simulink library "elvio"  (R2017a)
settings: Solver=VariableStepAuto  StartTime=0.0  StopTime=10.0  RelTol=1e-3
values from neighbouring files (symbols this model uses):
  Ts = 1    [dynorun.m]
  v = [v1;v2]    [elvio_plot_scatter.m]
undefined symbols (not defined in the file or in its folder): dm, elvio_tag_from, elvio_tag_goto, energy, F, Fmax, Fmin, Freq, m, request, speed, vcur
undefined symbols (not defined in the file): containers, torque
libraries: elvio x92, simulink x6
(part 1 of 2)
settings Model: Creator=elts2  LastModifiedBy=thomas

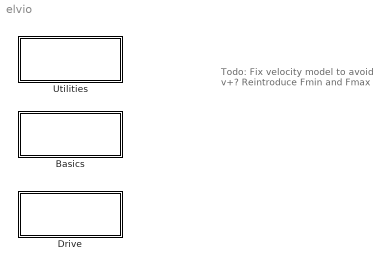
== system elvio ==
  note: Todo:
      | Fix velocity model to avoid v+?
      | Reintroduce Fmin and Fmax
  Basics : Subsystem
  Drive : Subsystem
  Utilities : Subsystem

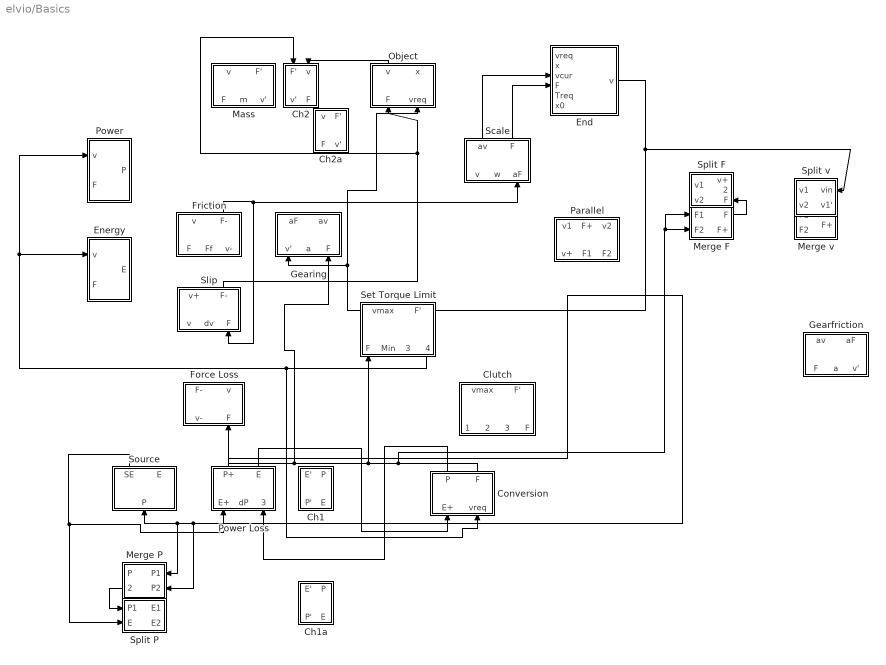
== system elvio/Basics ==
  Ch1 : Subsystem
  Ch1a : Subsystem
  Ch2 : Subsystem
  Ch2a : Subsystem
  Clutch : Subsystem
  Conversion : Subsystem
  End : Subsystem
  Energy : Subsystem
  Force Loss : Subsystem  mask{factor=0.1}
      mask prompts: factor "Loss Factor:"
  Friction : Subsystem
  Gearfriction : Subsystem
  Gearing : Subsystem
  Mass : Subsystem
  Merge F : Subsystem
  Merge P : Subsystem
  Merge v : Subsystem
  Object : Subsystem
  Parallel : Subsystem
  Power : Subsystem
  Power Loss : Subsystem
  Scale : Subsystem
  Set Torque Limit : Subsystem
  Slip : Subsystem
  Source : Subsystem
  Split F : Subsystem
  Split P : Subsystem
  Split v : Subsystem
  wires:
  Conversion/1(P) -> Power Loss/3(Preq)
  End/1(v) -> Split v/1(vin), Conversion/2(vreq), Power/1(v), Energy/1(v), Object/2(vreq), Gearing/1(v')
  Power Loss/1(P+) -> Merge P/2(P2), Merge P/1(P1), Source/1(P)
  Source/1(SE) -> Split P/2(E), Power Loss/1(E+)
  Conversion/2(F) -> Merge F/1(F1), Merge F/2(F2), Set Torque Limit/1(F), Force Loss/2(F), Gearing/3(F)
  Friction/2(F-) -> Scale/3(aF), Slip/3(F)
  Scale/1(av) -> End/3(vcur)
  Scale/2(F) -> End/4(F)
  Slip/2(F-) -> Ch2/1(F'), Object/1(F)
  Merge F/1(F) -> Split F/3(F)
  Power Loss/2(E) -> Conversion/1(E+)
  Object/1(v) -> Ch2/2(v)
  Merge P/2(P1'1) -> Split P/1(P1)

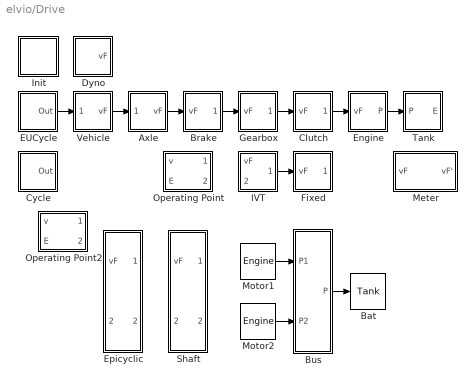
== system elvio/Drive ==
  Axle : Subsystem  InitFcn=|  mask{radius=0.3, ratio=4, factor=0.1, FromTag1=Vehicle1, GotoTag1=F}
      | elvio_tag_from([1]);
      | elvio_tag_goto([1]);
      mask prompts: radius "Tyre Radius (in m):"; ratio "Final Drive (ratio):"; factor "Loss Factor (factor):"; FromTag1 "Simulink:blkprm_prompts:FromGotoTag"; GotoTag1 "Simulink:blkprm_prompts:GotoTag"
      mask TypeOptions factor: Force Loss/factor
      mask TypeOptions FromTag1: From/GotoTag
      mask TypeOptions GotoTag1: Goto/GotoTag
  Bat : elvio/Drive/Tank  GotoTag1=F
  Brake : Subsystem  InitFcn=|  mask(Brake){Tbrake=5000, FromTag1=Vehicle1, GotoTag1=F}
      | elvio_tag_from([1]);
      | elvio_tag_goto([1]);
      mask prompts: Tbrake "Available Braking Torque (in Nm):"; FromTag1 "Simulink:blkprm_prompts:FromGotoTag"; GotoTag1 "Simulink:blkprm_prompts:GotoTag"
      mask help: This block adds braking torque when the powertrain cannot provide enough braking.
      mask TypeOptions FromTag1: From/GotoTag
      mask TypeOptions GotoTag1: Goto/GotoTag
  Bus : Subsystem  InitFcn=|  mask(DC Bus){GotoTag1=F, GotoTag2=E2, FromTag1=E}
      | elvio_tag_from([1]);
      | elvio_tag_goto([1 2]);
      mask prompts: GotoTag1 "Simulink:blkprm_prompts:GotoTag"; GotoTag2 "Simulink:blkprm_prompts:GotoTag"; FromTag1 "Simulink:blkprm_prompts:FromGotoTag"
      mask help: The DC bus connects two drives to one DC source.
      mask TypeOptions GotoTag1: Goto1/GotoTag
      mask TypeOptions GotoTag2: Goto2/GotoTag
      mask TypeOptions FromTag1: From1/GotoTag
  Clutch : Subsystem  InitFcn=|  mask(Clutch){speed=70, FromTag1=Vehicle1, GotoTag1=F}
      | elvio_tag_from([1]);
      | elvio_tag_goto([1]);
      mask prompts: speed "Minimum Speed (rad/s):"; FromTag1 "Simulink:blkprm_prompts:FromGotoTag"; GotoTag1 "Simulink:blkprm_prompts:GotoTag"
      mask help: This block enforces a minimal engine speed, simulating a slipping clutch when necessary.
      mask TypeOptions FromTag1: From/GotoTag
      mask TypeOptions GotoTag1: Goto/GotoTag
  Cycle : Subsystem  mask(Global Cycle){data=elvio_cycle_cadc_mw150()}
      mask prompts: data "Cycle:"
      mask help: This block generates one of the global cycles. Tolerances and gear information are reconstructed based on the approach used for NEDC.
      mask TypeOptions data: elvio_cycle_cadc_mw150() | elvio_cycle_cadc_rural() | elvio_cycle_cadc_urban() | elvio_cycle_cadc_urm150() | elvio_cycle_us_ftp75() | elvio_cycle_us_us06() | elvio_cycle_wltp_3b()
  Dyno : Subsystem  InitFcn=elvio_tag_from([1]);  mask{speed=speed, torque=torque, FromTag1=Dyno1}
      mask prompts: FromTag1 "Simulink:blkprm_prompts:FromGotoTag"
      mask TypeOptions FromTag1: From/GotoTag
  EUCycle : Subsystem  mask(European Cycle){data=elvio_cycle_nedc()}
      mask prompts: data "Cycle:"
      mask help: This block generates one of the European Cycles according to Regulation UNECE R83, including permissible tolerances and gear information.
      mask TypeOptions data: elvio_cycle_nedc() | elvio_cycle_ece15() | elvio_cycle_eudc()
  Engine : Subsystem  InitFcn=|  mask(Loss Model){Tmax=110, Tmin=0, Tfrict=16, Ploss=800, lossf=0.8, lossnorm=125e3, lossR=0.25, FromTag1=E, GotoTag1=F}
      | elvio_tag_from([1]);
      | elvio_tag_goto([1]);
      mask prompts: Tmax "Max Torque:"; Tmin "Min Torque:"; Tfrict "Friction Torque (Nm):"; Ploss "Power Loss (W):"; lossf "Loss Factor (factor):"; lossnorm "Square Loss Normal (W):"; lossR "Slip Loss (rad/Nms):"; FromTag1 "Simulink:blkprm_prompts:FromGotoTag"; GotoTag1 "Simulink:blkprm_prompts:GotoTag"
      mask help: A simple parametric engine or motor model based on 5 loss models.
      mask Help:
      | The five loss models are:
      |  * constant friction torque
      |  * constant power loss
      |  * constant efficiency loss
      |  * slip like loss (damping)
      |  * square of the power loss, defined using the nomalized power where the loss equalls the full power
      | 
      | To create a model with twice the torque, the friction, power loss, and square loss have to doubled, and the slip damping has to be halved.
      | 
      | To create a model with twice the speed, the power loss, the slip damping, and the square power have to be doubled.
      mask TypeOptions FromTag1: From/GotoTag
      mask TypeOptions GotoTag1: Goto/GotoTag
  Epicyclic : Subsystem  InitFcn=|  mask(Epicyclic Gearbox){a=0.3, FromTag1=E, FromTag2=F2, GotoTag1=F}
      | elvio_tag_from([1 2]);
      | elvio_tag_goto([1]);
      mask prompts: a "Sun to Ring Ratio (factor):"; FromTag1 "Simulink:blkprm_prompts:FromGotoTag"; FromTag2 "Simulink:blkprm_prompts:FromGotoTag"; GotoTag1 "Simulink:blkprm_prompts:GotoTag"
      mask help:
      | Model of an epicyclic gearbox (or velocity summing junction).
      |
      | It combines the speed of two prime movers, and splits the torque evenly according to the ratio.
      |
      | Rc is the relocity reference for the carrier vFc.
      mask TypeOptions FromTag1: From1/GotoTag
      mask TypeOptions FromTag2: From2/GotoTag
      mask TypeOptions GotoTag1: Goto/GotoTag
  Fixed : Subsystem  InitFcn=|  mask(Fixed Gear){gear=2, factor=0.1, FromTag1=E, GotoTag1=F}
      | elvio_tag_from([1]);
      | elvio_tag_goto([1]);
      mask prompts: gear "Gearing (ratio):"; factor "Loss Factor (factor):"; FromTag1 "Simulink:blkprm_prompts:FromGotoTag"; GotoTag1 "Simulink:blkprm_prompts:GotoTag"
      mask help: Model of a fixed gear with constant efficiency.
      mask TypeOptions factor: Force Loss/factor
      mask TypeOptions FromTag1: From/GotoTag
      mask TypeOptions GotoTag1: Goto/GotoTag
  Gearbox : Subsystem  InitFcn=|  mask(Manual Gearbox){gears=[4 2.5 1.8 1.2 0.9 0.9], factor=0.1, FromTag1=Gearbox1, GotoTag1=Brake1}
      | elvio_tag_from([1]);
      | elvio_tag_goto([1]);
      mask prompts: gears "Gears (vector):"; factor "Loss Factor (factor):"; FromTag1 "Simulink:blkprm_prompts:FromGotoTag"; GotoTag1 "Simulink:blkprm_prompts:GotoTag"
      mask help: This block is a manual gearbox. It applies to gear chosen by the cycle.
      mask TypeOptions factor: Force Loss/factor
      mask TypeOptions FromTag1: From/GotoTag
      mask TypeOptions GotoTag1: Goto/GotoTag
  IVT : Subsystem  InitFcn=|  mask{factor=0.1, FromTag1=E, GotoTag1=F}
      | elvio_tag_from([1]);
      | elvio_tag_goto([1]);
      mask prompts: factor "Loss Factor:"; FromTag1 "Simulink:blkprm_prompts:FromGotoTag"; GotoTag1 "Simulink:blkprm_prompts:GotoTag"
      mask TypeOptions factor: Force Loss/factor
      mask TypeOptions FromTag1: From/GotoTag
      mask TypeOptions GotoTag1: Goto/GotoTag
  Init : Subsystem  InitFcn=|  mask(Initialization Block){Ts0=1}
      | if ~exist('Ts')
      |     Ts = Ts0;
      | end
      | 
      | if ~exist('handle')
      |     handle = struct();
      | end
      mask prompts: Ts0 "Sample Time:"
      mask help: Initialize the Elvio library. This block sets the sampling time. It needs to be present in every Elvio model.
  Meter : Subsystem  InitFcn=|  mask(Energy Meter){FromTag1=E, GotoTag1=F}
      | elvio_tag_from([1]);
      | elvio_tag_goto([1]);
      mask prompts: FromTag1 "Simulink:blkprm_prompts:FromGotoTag"; GotoTag1 "Simulink:blkprm_prompts:GotoTag"
      mask help: Displays how much energy has flown through this connection so far, in J.
      mask TypeOptions FromTag1: From/GotoTag
      mask TypeOptions GotoTag1: Goto/GotoTag
  Motor1 : elvio/Drive/Engine  Tmax=60  Tmin=0  Tfrict=0.2  Ploss=100  lossf=0.01  lossnorm=2e6  lossR=0.05  FromTag1=E  GotoTag1=F
  Motor2 : elvio/Drive/Engine  Tmax=60  Tmin=-60  Tfrict=1  Ploss=200  lossf=0.01  lossnorm=1e6  lossR=0.1  FromTag1=E  GotoTag1=F
  Operating Point : Subsystem  mask{a=0.4, T=1000, Pk=0.5, Pbias=10e3, Pmin=5e3, vmin=100, vmax=400, Tmin=10, Tmax=80}
      mask prompts: a "Sun to Ring Ratio:"; T "SoC Time Constant:"; Pk "Power Gain:"; Pbias "Power Bias:"; Pmin "Power Minimum:"; vmin "Speed Minimum:"; vmax "Speed Maximum:"; Tmin "Torque Minimum:"; Tmax "Torque Maximum:"
  Operating Point2 : Subsystem  mask{a=0.4, T=1000, Preq=[0 5 5.001 60]*1e3, Pice=[0 0 6 50]*1e3, vopt=[0 100 100 500], Topt=[0 0 100 100]}
      mask prompts: a "Sun to Ring Ratio:"; T "SoC Time Constant:"; Preq "Requested Power:"; Pice "Engine Powor:"; vopt "Optimal Speed:"; Topt "Optimal Torque:"
  Shaft : Subsystem  InitFcn=|  mask(Mechanical Shaft){FromTag1=E, FromTag2=F2, GotoTag1=F}
      | elvio_tag_from([1 2]);
      | elvio_tag_goto([1]);
      mask prompts: FromTag1 "Simulink:blkprm_prompts:FromGotoTag"; FromTag2 "Simulink:blkprm_prompts:FromGotoTag"; GotoTag1 "Simulink:blkprm_prompts:GotoTag"
      mask help:
      | The shaft combines the torque of two prime movers at the same speed.
      |
      | R1 is the force reference for vF1, but it is subject to the available torque of vF1 and vF2.
      mask TypeOptions FromTag1: From1/GotoTag
      mask TypeOptions FromTag2: From2/GotoTag
      mask TypeOptions GotoTag1: Goto/GotoTag
  Tank : Subsystem  InitFcn=elvio_tag_goto([1]);  mask(Energy){GotoTag1=F}
      mask prompts: GotoTag1 "Simulink:blkprm_prompts:GotoTag"
      mask help: The fuel tank or the battery are modelled as an energy store, relative to the start of the simulation. The energy is measured in J, and it goes negative as energy is being used.
      mask TypeOptions GotoTag1: Goto/GotoTag
  Vehicle : Subsystem  InitFcn=elvio_tag_from([1]);  mask(Vehicle Body Model){m=1200, Froll=150, Aeff=0.4, n=[10 1], FromTag1=Vehicle1}
      mask prompts: m "Vehicle Mass (in kg):"; Froll "Tyre Friction (factor):"; Aeff "Aero Drag 0.5ρAef (in Ns²/m²):"; n "Number of Simulation (2d):"; FromTag1 "Simulink:blkprm_prompts:FromGotoTag"
      mask help: This block models the inertia and the aerodynamic drag and tyre rolling friction of a vehicle. It turns the cycle into a required tractive effort.
      mask TypeOptions FromTag1: From/GotoTag
  wires:
  Engine/1(P) -> Tank/1(P)
  Gearbox/1(vF') -> Clutch/1(vF)
  EUCycle/1(Out) -> Vehicle/1(vreq)
  Bus/1(P) -> Bat/1
  Motor1/1 -> Bus/1(P1)
  Motor2/1 -> Bus/2(P2)
  Brake/1(vF') -> Gearbox/1(vF)
  Clutch/1(vF') -> Engine/1(vF)
  IVT/1(vF') -> Fixed/1(vF)
  Axle/1(vF) -> Brake/1(vF)
  Vehicle/1(vF) -> Axle/1(vreq)

== system elvio/Utilities ==
  note: Testing
  Ch0 : Subsystem  mask{e=1e-6, e0=1}
      mask prompts: e "Relative Error:"; e0 "Initial Size:"
  Datafunction : Subsystem  mask{Cycle=NEDC, Data=[0 0 10 10 0 0]}
      mask prompts: Cycle "Driving Cycle:"; Data "Time Data:"
      mask init:
      | c=get_param(gcbh,'Cycle');
      | if c == "NEDC"
      |     set_param(gcbh,'Data','[0 0 10 10 0 0]');
      | end
      mask TypeOptions Cycle: NEDC | Artemis | FTP-75
  Display : Subsystem  StartFcn=h=elvio_display_start();  mask(Display the Input Value){}
      mask help: Todo: may display in the wrong blob? BUG
  Integrator : Subsystem  mask{Ts=Ts}
      mask prompts: Ts "Time Step:"
  Integrator+ : Subsystem  mask{Ts=Ts}
      mask prompts: Ts "Time Step:"
  Range : Subsystem
  Unit : Subsystem  mask(Constant value with units){Value=10, unitstr=rpm, unitmap=containers.Map({'rad/s','Hz','rpm','hrpm','krpm'},[1 2*pi 2*pi/60 2*pi/60*100 2*pi/60*1000])}
      mask prompts: Value "Simulink:blkprm_prompts:ConstConstValue"; unitmap "Unit map:"
      mask help:
      | This is a generic block for a value with units.
      |
      | The units can be configured with the field unitmap.
      mask TypeOptions Value: Constant/Value
      mask Display: disp('Value')
  Variants : Subsystem  Variant=on  VariantControl=Variant1  OverrideUsingVariant=Variant1

== system elvio/Basics/Ch1 ==
  E' : Inport
  P : Inport  Port=2
  Bus Selector1 : BusSelector  OutputSignals=P,info.w,info.x0
  Bus Selector3 : BusSelector  OutputSignals=energy
  Bus v : BusAssignment  AssignedSignals=P
  Ch0 : elvio/Utilities/Ch0  e=1e-6  e0=1
  Integrator : elvio/Utilities/Integrator  Ts=Ts
  Product : Product
  Terminator : Terminator
  P' : Outport
  E : Outport  Port=2
  wires:
  Product/1 -> Integrator/1
  E'/1 -> E/1, Bus Selector3/1
  Bus Selector1/3 -> Integrator/2  "<x0>"
  P/1 -> Bus Selector1/1, Bus v/1
  Bus Selector1/1 -> Bus v/2, Product/2  "<P>"
  Bus v/1 -> P'/1
  Bus Selector1/2 -> Product/1  "<w>"
  Integrator/1 -> Terminator/1
  Integrator/2 -> Ch0/1
  Bus Selector3/1 -> Ch0/2  "<energy>"

== system elvio/Basics/Ch1a ==
  E' : Inport
  P : Inport  Port=2
  Bus Selector1 : BusSelector  OutputSignals=P,info.w,info.x0
  Bus Selector3 : BusSelector  OutputSignals=energy
  Ch0 : elvio/Utilities/Ch0  e=1e-6  e0=1
  Integrator : elvio/Utilities/Integrator  Ts=Ts
  Product : Product
  Terminator : Terminator
  P' : Outport
  E : Outport  Port=2
  wires:
  Bus Selector3/1 -> Ch0/2  "<energy>"
  Integrator/2 -> Ch0/1
  Integrator/1 -> Terminator/1
  Bus Selector1/2 -> Product/2  "<w>"
  Bus Selector1/1 -> Product/1  "<P>"
  P/1 -> P'/1, Bus Selector1/1
  Bus Selector1/3 -> Integrator/2  "<x0>"
  E'/1 -> Bus Selector3/1, E/1
  Product/1 -> Integrator/1

== system elvio/Basics/Ch2 ==
  F' : Inport
  v : Inport  Port=2
  Bus Selector1 : BusSelector  OutputSignals=info.x0
  Bus Selector2 : BusSelector  OutputSignals=Freq
  Bus Selector3 : BusSelector  OutputSignals=F
  Bus Selector4 : BusSelector  OutputSignals=energy
  Ch0 : elvio/Utilities/Ch0  e=1e-6  e0=1
  Check Static Range : simulink/Model Verification/Check  Static Range  Description=-1e-10 <= u <= 1e-10  max=1e-10  max_included=on  min=-1e-10  min_included=on  enabled=on  stopWhenAssertionFail=on  export=off  icon=graphic
      settings: SourceProductName=Simulink  SourceProductBaseCode=SL
  Integrator : elvio/Utilities/Integrator  Ts=Ts
  Power : elvio/Basics/Power
  Sum2 : Sum  Inputs=+-
  Terminator : Terminator
  v' : Outport
  F : Outport  Port=2
  wires:
  Bus Selector3/1 -> Power/2, Sum2/2  "<F>"
  Power/1 -> Integrator/1
  F'/1 -> F/1, Bus Selector4/1, Bus Selector3/1
  Bus Selector1/1 -> Integrator/2  "<x0>"
  v/1 -> Bus Selector1/1, Power/1, Bus Selector2/1, v'/1
  Bus Selector2/1 -> Sum2/1  "<Freq>"
  Sum2/1 -> Check Static Range/1
  Integrator/1 -> Terminator/1
  Integrator/2 -> Ch0/1
  Bus Selector4/1 -> Ch0/2  "<energy>"

== system elvio/Basics/Ch2a ==
  v : Inport
  F' : Inport  Port=2
  Bus Selector1 : BusSelector  OutputSignals=info.x0
  Bus Selector2 : BusSelector  OutputSignals=Freq
  Bus Selector3 : BusSelector  OutputSignals=F
  Bus Selector4 : BusSelector  OutputSignals=energy
  Ch0 : elvio/Utilities/Ch0  e=1e-6  e0=1
  Check Static Range : simulink/Model Verification/Check  Static Range  Description=-1e-10 <= u <= 1e-10  max=1e-10  max_included=on  min=-1e-10  min_included=on  enabled=on  stopWhenAssertionFail=on  export=off  icon=graphic
      settings: SourceProductName=Simulink  SourceProductBaseCode=SL
  Integrator : elvio/Utilities/Integrator  Ts=Ts
  Power : elvio/Basics/Power
  Sum2 : Sum  Inputs=+-
  Terminator : Terminator
  F : Outport
  v' : Outport  Port=2
  wires:
  Bus Selector4/1 -> Ch0/2  "<energy>"
  Integrator/2 -> Ch0/1
  Integrator/1 -> Terminator/1
  Sum2/1 -> Check Static Range/1
  Bus Selector2/1 -> Sum2/1  "<Freq>"
  v/1 -> Bus Selector1/1, v'/1, Power/1, Bus Selector2/1
  Bus Selector1/1 -> Integrator/2  "<x0>"
  F'/1 -> Bus Selector3/1, F/1, Bus Selector4/1
  Power/1 -> Integrator/1
  Bus Selector3/1 -> Sum2/2, Power/2  "<F>"

== system elvio/Basics/Clutch ==
  note: Todo
  vreq : Inport
  Fmax : Inport  Port=2
  Fmin : Inport  Port=3
  F : Inport  Port=4
  Bus Selector1 : BusSelector  OutputSignals=Freq
  Bus F : BusAssignment  AssignedSignals=Fmax,Fmin,F
  Bus v : BusAssignment  AssignedSignals=Freq
  Range : Subsystem
  vmax : Outport
  F' : Outport  Port=2
  wires:
  F/1 -> Bus F/1
  Range/1(Out) -> Bus F/4, Bus v/2  "F"
  Bus Selector1/1 -> Range/2(In)  "<Freq>"
  vreq/1 -> Bus v/1, Bus Selector1/1
  Bus v/1 -> vmax/1
  Fmin/1 -> Range/3(Min), Bus F/3  "Fmin"
  Fmax/1 -> Range/1(Max), Bus F/2
  Bus F/1 -> F'/1

== system elvio/Basics/Conversion ==
  E+ : Inport
  vreq : Inport  Port=2
  Bias1 : Bias  Bias=1e10
  Bias2 : Bias  Bias=-1e10
  Bus Creator1 : BusCreator  Inputs=8
  Bus Selector : BusSelector  OutputSignals=info.x0,Freq
  Bus Selector3 : BusSelector  OutputSignals=energy
  Constant{4..7} (4 alike) : Constant  Value=0
  Power : Subsystem
  unity : Gain
  zero : Gain  Gain=0
  P : Outport
  F : Outport  Port=2
  wires:
  Power/1(P) -> P/1
  Constant7/1 -> Bus Creator1/7  "power"
  Constant5/1 -> Bus Creator1/5  "dm"
  Bus Selector/2 -> unity/1, Power/2(F)  "<Freq>"
  Bus Creator1/1 -> F/1
  Constant6/1 -> Bus Creator1/6  "weight"
  Constant4/1 -> Bus Creator1/4  "m"
  vreq/1 -> Power/1(v), Bus Selector/1
  unity/1 -> Bus Creator1/1  "F"
  E+/1 -> Bus Selector3/1
  Bus Selector3/1 -> Bus Creator1/8  "<energy>"
  zero/1 -> Bias2/1, Bias1/1
  Bias2/1 -> Bus Creator1/3  "Fmin"
  Bus Selector/1 -> zero/1  "<x0>"
  Bias1/1 -> Bus Creator1/2  "Fmax"

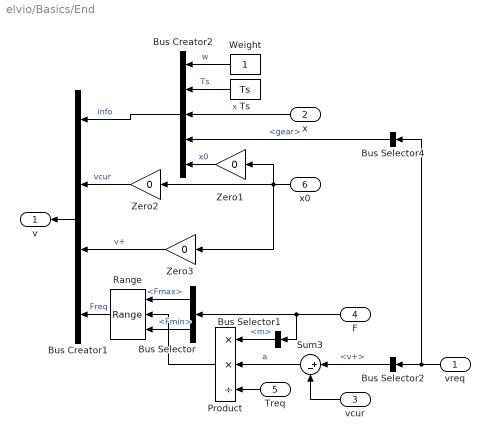
== system elvio/Basics/End ==
  vreq : Inport  Unit=m/s
  x : Inport  Port=2  Unit=m/s
  vcur : Inport  Port=3  Unit=m/s
  F : Inport  Port=4  Unit=m/s
  Treq : Inport  Port=5  Unit=m/s
  x0 : Inport  Port=6  Unit=m/s
  Bus Creator1 : BusCreator  Inputs=4
  Bus Creator2 : BusCreator  Inputs=5
  Bus Selector : BusSelector  OutputSignals=Fmax,Fmin
  Bus Selector1 : BusSelector  OutputSignals=m
  Bus Selector2 : BusSelector  OutputSignals=v+
  Bus Selector4 : BusSelector  OutputSignals=gear
  Product : Product  Inputs=**/
  Range : elvio/Utilities/Range
  Sum3 : Sum  Inputs=|+-
  Ts : Constant  Value=Ts
  Weight : Constant
  Zero1 : Gain  Gain=0
  Zero2 : Gain  Gain=0
  Zero3 : Gain  Gain=0
  v : Outport
  wires:
  x/1 -> Bus Creator2/3  "x"
  Weight/1 -> Bus Creator2/1  "w"
  Bus Creator1/1 -> v/1
  F/1 -> Bus Selector/1, Bus Selector1/1
  Bus Creator2/1 -> Bus Creator1/1  "info"
  Range/1 -> Bus Creator1/4  "Freq"
  Sum3/1 -> Product/2  "a"
  Zero2/1 -> Bus Creator1/2  "vcur"
  Zero3/1 -> Bus Creator1/3  "v+"
  vcur/1 -> Sum3/2
  Treq/1 -> Product/3
  x0/1 -> Zero2/1, Zero3/1, Zero1/1
  Zero1/1 -> Bus Creator2/5  "x0"
  Ts/1 -> Bus Creator2/2  "Ts"
  Bus Selector1/1 -> Product/1  "<m>"
  Bus Selector/1 -> Range/1  "<Fmax>"
  Bus Selector/2 -> Range/3  "<Fmin>"
  Product/1 -> Range/2
  Bus Selector4/1 -> Bus Creator2/4  "<gear>"
  Bus Selector2/1 -> Sum3/1  "<v+>"
  vreq/1 -> Bus Selector4/1, Bus Selector2/1

== system elvio/Basics/Energy ==
  v : Inport
  F : Inport  Port=2
  Bus Selector : BusSelector  OutputSignals=info.x0
  Integrator : elvio/Utilities/Integrator  Ts=Ts
  Power : elvio/Basics/Power
  Terminator : Terminator
  E : Outport
  wires:
  v/1 -> Bus Selector/1, Power/1
  Power/1 -> Integrator/1
  F/1 -> Power/2
  Bus Selector/1 -> Integrator/2  "<x0>"
  Integrator/1 -> Terminator/1
  Integrator/2 -> E/1

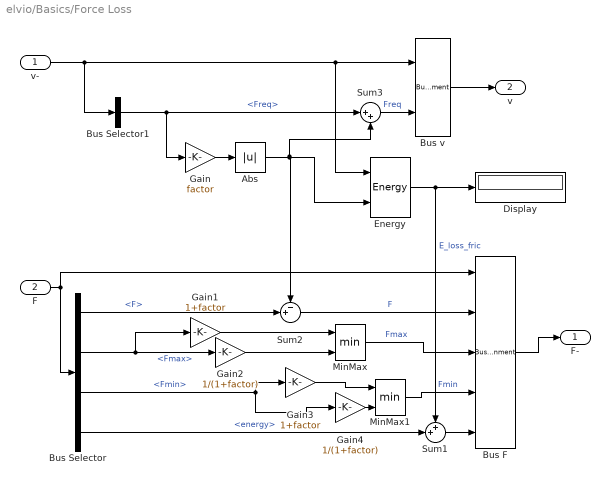
== system elvio/Basics/Force Loss ==
  v- : Inport
  F : Inport  Port=2
  Abs : Abs
  Bus Selector : BusSelector  OutputSignals=F,Fmax,Fmin,energy
  Bus Selector1 : BusSelector  OutputSignals=Freq
  Bus F : BusAssignment  AssignedSignals=F,Fmax,Fmin,energy
  Bus v : BusAssignment  AssignedSignals=Freq
  Display : Display
  Energy : elvio/Basics/Energy
  Gain : Gain  Gain=factor
  Gain1 : Gain  Gain=1+factor
  Gain2 : Gain  Gain=1/(1+factor)
  Gain3 : Gain  Gain=1+factor
  Gain4 : Gain  Gain=1/(1+factor)
  MinMax : MinMax  Inputs=2
  MinMax1 : MinMax  Inputs=2
  Sum1 : Sum  Inputs=++|
  Sum2 : Sum  Inputs=-+|
  Sum3 : Sum  Inputs=|++
  F- : Outport
  v : Outport  Port=2
  wires:
  MinMax/1 -> Bus F/3  "Fmax"
  MinMax1/1 -> Bus F/4  "Fmin"
  Bus Selector/3 -> Gain4/1, Gain3/1  "<Fmin>"
  Bus Selector/2 -> Gain1/1, Gain2/1  "<Fmax>"
  Sum1/1 -> Bus F/5
  Bus Selector/1 -> Sum2/2  "<F>"
  F/1 -> Bus F/1, Bus Selector/1
  Bus v/1 -> v/1
  Bus F/1 -> F-/1
  Sum2/1 -> Bus F/2  "F"
  Bus Selector1/1 -> Gain/1, Sum3/1  "<Freq>"
  Sum3/1 -> Bus v/2  "Freq"
  v-/1 -> Energy/1, Bus v/1, Bus Selector1/1
  Energy/1 -> Display/1, Sum1/1  "E_loss_fric"
  Gain/1 -> Abs/1
  Abs/1 -> Sum3/2, Sum2/1, Energy/2
  Gain2/1 -> MinMax/2
  Gain1/1 -> MinMax/1
  Gain4/1 -> MinMax1/2
  Gain3/1 -> MinMax1/1
  Bus Selector/4 -> Sum1/2  "<energy>"

== system elvio/Basics/Friction ==
  F : Inport
  Ff : Inport  Port=2
  v- : Inport  Port=3
  Bus Selector : BusSelector  OutputSignals=F,Fmax,Fmin,energy
  Bus Selector1 : BusSelector  OutputSignals=Freq
  Bus F : BusAssignment  AssignedSignals=F,Fmax,Fmin,energy
  Bus v : BusAssignment  AssignedSignals=Freq
  Energy : elvio/Basics/Energy
  Sum1 : Sum  Inputs=++|
  Sum2 : Sum  Inputs=-+|
  Sum3 : Sum  Inputs=|++
  Sum4 : Sum  Inputs=-+|
  Sum5 : Sum  Inputs=-+|
  v : Outport
  F- : Outport  Port=2
  wires:
  Energy/1 -> Sum1/1  "E_loss_fric"
  v-/1 -> Energy/1, Bus Selector1/1, Bus v/1
  Sum3/1 -> Bus v/2  "Freq"
  Bus Selector1/1 -> Sum3/1  "<Freq>"
  Sum2/1 -> Bus F/2  "F"
  Bus F/1 -> F-/1
  Ff/1 -> Sum4/1, Sum5/1, Energy/2, Sum2/1, Sum3/2
  Bus v/1 -> v/1
  F/1 -> Bus Selector/1, Bus F/1
  Bus Selector/1 -> Sum2/2  "<F>"
  Sum1/1 -> Bus F/5
  Bus Selector/4 -> Sum1/2  "<energy>"
  Bus Selector/2 -> Sum4/2  "<Fmax>"
  Bus Selector/3 -> Sum5/2  "<Fmin>"
  Sum5/1 -> Bus F/4  "Fmin"
  Sum4/1 -> Bus F/3  "Fmax"

== system elvio/Basics/Gearfriction ==
  F : Inport
  a : Inport  Port=2
  v' : Inport  Port=3
  Bias : Bias  Bias=1
  Bus Selector : BusSelector  OutputSignals=F,Fmax,Fmin,m,dm
  Bus Selector1 : BusSelector  OutputSignals=Freq
  Bus F : BusAssignment  AssignedSignals=F,Fmax,Fmin,m,dm
  Bus v : BusAssignment  AssignedSignals=Freq
  Minus : Gain  Gain=-1
  Product1 : Product
  Product2 : Product  Inputs=/*
  Product3 : Product
  Product8 : Product  Inputs=/*
  Todo : Gain
  av : Outport
  aF : Outport  Port=2
  wires:
  Bus Selector/3 -> Product2/2  "<Fmin>"
  Product2/1 -> Bus F/4  "Fmin"
  Bus Selector/2 -> Product1/2  "<Fmax>"
  Product1/1 -> Bus F/3  "Fmax"
  Bus Selector1/1 -> Product8/2  "<Freq>"
  Product3/1 -> Bus F/2  "F"
  a/1 -> Minus/1
  Bus Selector/4 -> Bus F/5  "<m>"
  Bus Selector/1 -> Product3/2  "<F>"
  Bus Selector/5 -> Todo/1  "<dm>"
  Bus v/1 -> av/1
  Product8/1 -> Bus v/2  "Freq"
  F/1 -> Bus F/1, Bus Selector/1
  v'/1 -> Bus v/1, Bus Selector1/1
  Todo/1 -> Bus F/6
  Bus F/1 -> aF/1
  Bias/1 -> Product3/1, Product2/1, Product1/1, Product8/1
  Minus/1 -> Bias/1

== system elvio/Basics/Gearing ==
  v' : Inport
  a : Inport  Port=2
  F : Inport  Port=3
  Bus Selector : BusSelector  OutputSignals=F,Fmax,Fmin,m,dm
  Bus Selector1 : BusSelector  OutputSignals=vcur,v+,Freq
  Bus F : BusAssignment  AssignedSignals=F,Fmax,Fmin,m,dm
  Bus v : BusAssignment  AssignedSignals=vcur,v+,Freq
  Product{1..3,5,13} (5 alike) : Product
  Product7 : Product  Inputs=***
  Product8 : Product  Inputs=/*
  Todo : Gain
  aF : Outport
  av : Outport  Port=2
  wires:
  Bus F/1 -> aF/1
  Todo/1 -> Bus F/6
  v'/1 -> Bus Selector1/1, Bus v/1
  Bus Selector1/2 -> Product13/2  "<v+>"
  Product13/1 -> Bus v/3  "v+"
  Bus Selector1/1 -> Product5/2  "<vcur>"
  F/1 -> Bus F/1, Bus Selector/1
  Product8/1 -> Bus v/4  "Freq"
  Bus v/1 -> av/1
  Bus Selector/5 -> Todo/1  "<dm>"
  Bus Selector/1 -> Product3/2  "<F>"
  Bus Selector/4 -> Product7/3  "<m>"
  a/1 -> Product5/1, Product13/1, Product8/1, Product3/1, Product1/1, Product7/1, Product7/2, Product2/1
  Product7/1 -> Bus F/5  "m"
  Product3/1 -> Bus F/2  "F"
  Bus Selector1/3 -> Product8/2  "<Freq>"
  Product5/1 -> Bus v/2  "vcur"
  Product1/1 -> Bus F/3  "Fmax"
  Bus Selector/2 -> Product1/2  "<Fmax>"
  Product2/1 -> Bus F/4  "Fmin"
  Bus Selector/3 -> Product2/2  "<Fmin>"

== system elvio/Basics/Mass ==
  F : Inport
  m : Inport  Port=2
  v' : Inport  Port=3
  Bus Assignment : BusAssignment  AssignedSignals=m
  Bus Selector : BusSelector  OutputSignals=m
  Sum : Sum  Inputs=|++
  v : Outport
  F' : Outport  Port=2
  wires:
  m/1 -> Sum/2
  Sum/1 -> Bus Assignment/2  "m"
  Bus Selector/1 -> Sum/1  "<m>"
  v'/1 -> v/1
  F/1 -> Bus Assignment/1, Bus Selector/1
  Bus Assignment/1 -> F'/1

== system elvio/Basics/Merge F ==
  F1 : Inport
  F2 : Inport  Port=2
  Bus Creator : BusCreator  Inputs=8
  Bus Creator1 : BusCreator  Inputs=2
  Bus Selector : BusSelector  OutputSignals=F,Fmax,Fmin,m,dm,weight,power,energy
  Bus Selector2 : BusSelector  OutputSignals=F,Fmax,Fmin,m,dm,weight,power,energy
  Sum{,1..7} (8 alike) : Sum  Inputs=|++
  F : Outport
  F+ : Outport  Port=2
  wires:
  Bus Selector/6 -> Sum3/1  "<weight>"
  Bus Selector/4 -> Sum1/1  "<m>"
  Bus Selector/5 -> Sum2/1  "<dm>"
  Bus Selector/7 -> Sum4/1  "<power>"
  F1/1 -> Bus Creator1/1, Bus Selector/1  "F1"
  Bus Selector/1 -> Sum/1  "<F>"
  F2/1 -> Bus Creator1/2, Bus Selector2/1  "F2"
  Bus Creator/1 -> F+/1
  Sum/1 -> Bus Creator/1  "F"
  Sum2/1 -> Bus Creator/5  "dm"
  Bus Selector2/5 -> Sum2/2  "<dm>"
  Bus Selector2/1 -> Sum/2  "<F>"
  Bus Selector2/7 -> Sum4/2  "<power>"
  Sum4/1 -> Bus Creator/7  "power"
  Sum6/1 -> Bus Creator/8  "energy"
  Sum1/1 -> Bus Creator/4  "m"
  Sum3/1 -> Bus Creator/6  "weight"
  Bus Selector/8 -> Sum6/1  "<energy>"
  Bus Selector2/6 -> Sum3/2  "<weight>"
  Bus Selector2/8 -> Sum6/2  "<energy>"
  Bus Selector2/4 -> Sum1/2  "<m>"
  Bus Selector/3 -> Sum7/1  "<Fmin>"
  Sum7/1 -> Bus Creator/3  "Fmin"
  Bus Selector/2 -> Sum5/1  "<Fmax>"
  Sum5/1 -> Bus Creator/2  "Fmax"
  Bus Selector2/2 -> Sum5/2  "<Fmax>"
  Bus Selector2/3 -> Sum7/2  "<Fmin>"
  Bus Creator1/1 -> F/1

== system elvio/Basics/Merge P ==
  P1 : Inport
  P2 : Inport  Port=2
  Bus Assignment : BusAssignment  AssignedSignals=P
  Bus Selector1 : BusSelector  OutputSignals=P
  Bus Selector2 : BusSelector  OutputSignals=P
  Sum : Sum  Inputs=|++
  P : Outport
  P1'1 : Outport  Port=2
  wires:
  P2/1 -> Bus Selector1/1
  P1/1 -> P1'1/1, Bus Assignment/1, Bus Selector2/1
  Bus Selector2/1 -> Sum/1  "<P>"
  Sum/1 -> Bus Assignment/2
  Bus Selector1/1 -> Sum/2  "<P>"
  Bus Assignment/1 -> P/1

== system elvio/Basics/Merge v ==
  note: Todo
  F1 : Inport
  F2 : Inport  Port=2
  Bus Creator : BusCreator  Inputs=8
  Bus Selector : BusSelector  OutputSignals=F,Fmax,Fmin,m,dm,weight,power,energy
  Bus Selector2 : BusSelector  OutputSignals=F,Fmax,Fmin,m,dm,weight,power,energy
  Highest Min : MinMax  Function=max  Inputs=2
  Lowest Max : MinMax  Inputs=2
  Sum{1..4,6} (5 alike) : Sum  Inputs=|++
  Terminator : Terminator
  F+ : Outport
  wires:
  Bus Selector2/3 -> Highest Min/2  "<Fmin>"
  Bus Selector2/2 -> Lowest Max/2  "<Fmax>"
  Lowest Max/1 -> Bus Creator/2  "Fmax"
  Bus Selector/2 -> Lowest Max/1  "<Fmax>"
  Highest Min/1 -> Bus Creator/3  "Fmin"
  Bus Selector/3 -> Highest Min/1  "<Fmin>"
  Bus Selector2/4 -> Sum1/2  "<m>"
  Bus Selector2/8 -> Sum6/2  "<energy>"
  Bus Selector2/6 -> Sum3/2  "<weight>"
  Bus Selector/8 -> Sum6/1  "<energy>"
  Sum3/1 -> Bus Creator/6  "weight"
  Sum1/1 -> Bus Creator/4  "m"
  Sum6/1 -> Bus Creator/8  "energy"
  Sum4/1 -> Bus Creator/7  "power"
  Bus Selector2/7 -> Sum4/2  "<power>"
  Bus Selector2/5 -> Sum2/2  "<dm>"
  Sum2/1 -> Bus Creator/5  "dm"
  Bus Creator/1 -> F+/1
  F2/1 -> Bus Selector2/1
  Bus Selector/1 -> Bus Creator/1  "<F>"
  F1/1 -> Bus Selector/1
  Bus Selector/7 -> Sum4/1  "<power>"
  Bus Selector/5 -> Sum2/1  "<dm>"
  Bus Selector/4 -> Sum1/1  "<m>"
  Bus Selector/6 -> Sum3/1  "<weight>"
  Bus Selector2/1 -> Terminator/1  "<F>"

== system elvio/Basics/Object ==
  note: Todo
  F : Inport
  vreq : Inport  Port=2
  Bus Selector : BusSelector  OutputSignals=info.w,info.x0
  Bus Selector2 : BusSelector  OutputSignals=F,m,dm,energy
  Bus v : BusAssignment  AssignedSignals=vcur,v+
  Check Static Range : simulink/Model Verification/Check  Static Range  Description=-1e-3 <= u <= 1e-3  max=1e-3  max_included=on  min=-1e-3  min_included=on  enabled=on  stopWhenAssertionFail=on  export=off  icon=graphic
      settings: SourceProductName=Simulink  SourceProductBaseCode=SL
  Display : Display
  Division : Product  Inputs=*/
  Position : elvio/Utilities/Integrator  Ts=Ts
  Product : Product  Inputs=****
  Speed : elvio/Utilities/Integrator  Ts=Ts
  Sum : Sum  Inputs=|++
  Terminator2 : Terminator
  Todo : Terminator
  half : Gain  Gain=0.5
  v : Outport
  x : Outport  Port=2
  wires:
  vreq/1 -> Bus Selector/1, Bus v/1
  Bus Selector2/2 -> Product/3, Division/2  "<m>"
  Speed/1 -> Position/1, Bus v/2  "vcur"
  Division/1 -> Speed/1  "a"
  Product/1 -> half/1
  Bus Selector2/1 -> Division/1  "<F>"
  F/1 -> Bus Selector2/1
  half/1 -> Sum/1  "E_kin"
  Bus Selector2/3 -> Todo/1  "<dm>"
  Bus v/1 -> v/1
  Bus Selector/1 -> Product/4  "<w>"
  Position/2 -> x/1
  Position/1 -> Terminator2/1
  Speed/2 -> Product/2, Product/1, Bus v/3
  Bus Selector/2 -> Position/2, Speed/2  "<x0>"
  Bus Selector2/4 -> Sum/2  "<energy>"
  Sum/1 -> Check Static Range/1, Display/1

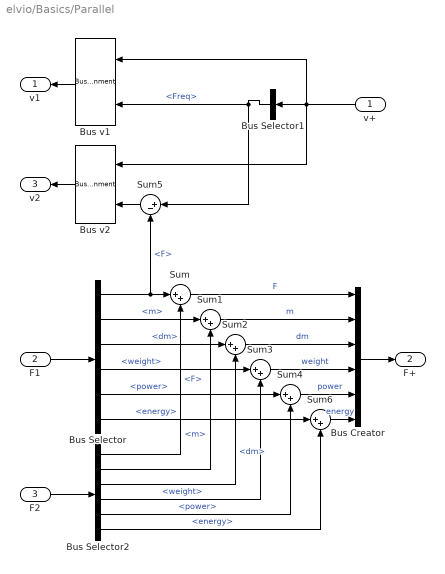
== system elvio/Basics/Parallel ==
  v+ : Inport
  F1 : Inport  Port=2
  F2 : Inport  Port=3
  Bus Creator : BusCreator  Inputs=6
  Bus Selector : BusSelector  OutputSignals=F,m,dm,weight,power,energy
  Bus Selector1 : BusSelector  OutputSignals=Freq
  Bus Selector2 : BusSelector  OutputSignals=F,m,dm,weight,power,energy
  Bus v1 : BusAssignment  AssignedSignals=Freq
  Bus v2 : BusAssignment  AssignedSignals=Freq
  Sum{,1..4,6} (6 alike) : Sum  Inputs=|++
  Sum5 : Sum  Inputs=|+-
  v1 : Outport
  F+ : Outport  Port=2
  v2 : Outport  Port=3
  wires:
  F1/1 -> Bus Selector/1
  Bus v1/1 -> v1/1
  Bus Selector1/1 -> Bus v1/2, Sum5/1  "<Freq>"
  Bus v2/1 -> v2/1
  v+/1 -> Bus v1/1, Bus v2/1, Bus Selector1/1
  Bus Selector/4 -> Sum3/1  "<weight>"
  Bus Selector/3 -> Sum2/1  "<dm>"
  Bus Selector/5 -> Sum4/1  "<power>"
  Bus Selector/2 -> Sum1/1  "<m>"
  Bus Selector/1 -> Sum5/2, Sum/1  "<F>"
  F2/1 -> Bus Selector2/1
  Bus Selector2/1 -> Sum/2  "<F>"
  Bus Selector2/2 -> Sum1/2  "<m>"
  Bus Selector2/3 -> Sum2/2  "<dm>"
  Bus Selector2/4 -> Sum3/2  "<weight>"
  Bus Selector2/5 -> Sum4/2  "<power>"
  Sum/1 -> Bus Creator/1  "F"
  Sum1/1 -> Bus Creator/2  "m"
  Sum2/1 -> Bus Creator/3  "dm"
  Sum3/1 -> Bus Creator/4  "weight"
  Sum4/1 -> Bus Creator/5  "power"
  Bus Creator/1 -> F+/1
  Sum5/1 -> Bus v2/2
  Sum6/1 -> Bus Creator/6  "energy"
  Bus Selector2/6 -> Sum6/2  "<energy>"
  Bus Selector/6 -> Sum6/1  "<energy>"

== system elvio/Basics/Power ==
  v : Inport
  F : Inport  Port=2
  Bus Selector2 : BusSelector  OutputSignals=vcur,v+,info.w
  Product : Product  Inputs=***
  Sum4 : Sum  Inputs=++|
  half : Gain  Gain=0.5
  P : Outport
  wires:
  half/1 -> P/1
  Bus Selector2/3 -> Product/2  "<w>"
  Bus Selector2/1 -> Sum4/1  "<vcur>"
  v/1 -> Bus Selector2/1
  Product/1 -> half/1
  Sum4/1 -> Product/1
  F/1 -> Product/3
  Bus Selector2/2 -> Sum4/2  "<v+>"

== system elvio/Basics/Power Loss ==
  E+ : Inport
  dP : Inport  Port=2
  Preq : Inport  Port=3
  Bus Selector1 : BusSelector  OutputSignals=P,info.w,info.x0
  Bus Selector3 : BusSelector  OutputSignals=energy
  Bus E : BusAssignment  AssignedSignals=energy
  Bus v : BusAssignment  AssignedSignals=P
  Integrator : elvio/Utilities/Integrator  Ts=Ts
  Product : Product
  Sum1 : Sum  Inputs=++|
  Sum3 : Sum  Inputs=|++
  Terminator : Terminator
  P+ : Outport
  E : Outport  Port=2
  wires:
  Integrator/2 -> Sum1/1  "E_power_loss"
  Product/1 -> Integrator/1
  Bus Selector1/2 -> Product/1  "<w>"
  Bus v/1 -> P+/1
  Bus Selector1/1 -> Sum3/1  "<P>"
  Sum3/1 -> Bus v/2  "Freq"
  dP/1 -> Sum3/2, Product/2
  Preq/1 -> Bus v/1, Bus Selector1/1
  Bus Selector1/3 -> Integrator/2  "<x0>"
  E+/1 -> Bus Selector3/1, Bus E/1
  Sum1/1 -> Bus E/2
  Bus E/1 -> E/1
  Bus Selector3/1 -> Sum1/2  "<energy>"
  Integrator/1 -> Terminator/1

== system elvio/Basics/Scale ==
  note: Todo: fix this block
  v : Inport
  w : Inport  Port=2
  aF : Inport  Port=3
  Bias : Bias  Bias=-1
  Bus Selector : BusSelector  OutputSignals=F,energy
  Bus Selector1 : BusSelector  OutputSignals=info.w
  Bus Selector2 : BusSelector  OutputSignals=P
  Bus Selector3 : BusSelector  OutputSignals=info.x0
  Bus F : BusAssignment  AssignedSignals=energy
  Bus v : BusAssignment  AssignedSignals=info.w
  Display : Display
  Integrator : elvio/Utilities/Integrator  Ts=Ts
  Power : Subsystem
  Product1 : Product
  Product2 : Product
  Sum : Sum  Inputs=++|
  av : Outport
  F : Outport  Port=2
  wires:
  Integrator/1 -> Sum/1, Display/1  "E_power"
  Bus Selector3/1 -> Integrator/2  "<x0>"
  Product2/1 -> Integrator/1  "E_power"
  Bias/1 -> Product2/1
  w/1 -> Product1/2, Bias/1
  Bus Selector2/1 -> Product2/2  "<P>"
  Bus Selector/1 -> Power/2(F)  "<F>"
  v/1 -> Bus v/1, Bus Selector1/1, Power/1(v), Bus Selector3/1
  Power/1(P) -> Bus Selector2/1
  Product1/1 -> Bus v/2  "vcur"
  Bus v/1 -> av/1
  Bus Selector1/1 -> Product1/1  "<w>"
  aF/1 -> Bus Selector/1, Bus F/1
  Bus F/1 -> F/1
  Sum/1 -> Bus F/2
  Bus Selector/2 -> Sum/2  "<energy>"

== system elvio/Basics/Set Torque Limit ==
  F : Inport
  Min : Inport  Port=2
  Max : Inport  Port=3
  vreq : Inport  Port=4
  Bus Selector : BusSelector  OutputSignals=Freq
  Bus Selector1 : BusSelector  OutputSignals=Fmax,Fmin
  Bus F : BusAssignment  AssignedSignals=Fmax,Fmin
  Bus v : BusAssignment  AssignedSignals=Freq
  Highest Min : MinMax  Function=max  Inputs=2
  Lowest Max : MinMax  Inputs=2
  Range : elvio/Utilities/Range
  vmax : Outport
  F' : Outport  Port=2
  wires:
  F/1 -> Bus Selector1/1, Bus F/1
  Bus v/1 -> vmax/1
  vreq/1 -> Bus Selector/1, Bus v/1
  Range/1 -> Bus v/2
  Bus Selector/1 -> Range/2  "<Freq>"
  Bus F/1 -> F'/1
  Lowest Max/1 -> Range/1, Bus F/2
  Highest Min/1 -> Range/3, Bus F/3
  Bus Selector1/1 -> Lowest Max/2  "<Fmax>"
  Bus Selector1/2 -> Highest Min/2  "<Fmin>"
  Max/1 -> Lowest Max/1
  Min/1 -> Highest Min/1

== system elvio/Basics/Slip ==
  v : Inport
  dv : Inport  Port=2
  F : Inport  Port=3
  Bus Selector : BusSelector  OutputSignals=F
  Bus Selector1 : BusSelector  OutputSignals=v+
  Bus Selector2 : BusSelector  OutputSignals=info.w
  Bus v : BusAssignment  AssignedSignals=vcur,v+
  Display : Display
  Integrator : elvio/Utilities/Integrator  Ts=Ts
  Product : Product  Inputs=***
  Sum5 : Sum  Inputs=|++
  Terminator : Terminator
  Unit Delay : UnitDelay  SampleTime=abs(Ts)
  half : Gain  Gain=0.5
  v+ : Outport
  F- : Outport  Port=2
  wires:
  Bus Selector2/1 -> Product/1  "<w>"
  v/1 -> Bus v/1, Bus Selector2/1, Bus Selector1/1
  half/1 -> Integrator/1
  Bus Selector/1 -> Product/3  "<F>"
  Integrator/2 -> Display/1  "E_loss_slip"
  Product/1 -> half/1
  dv/1 -> Sum5/2, Product/2
  Integrator/1 -> Terminator/1
  Sum5/1 -> Unit Delay/1, Bus v/3
  Bus Selector1/1 -> Sum5/1  "<v+>"
  F/1 -> Bus Selector/1, F-/1
  Bus v/1 -> v+/1
  Unit Delay/1 -> Bus v/2

== system elvio/Basics/Source ==
  P : Inport
  Bias : Bias  Bias=1e-10
  Bus Creator : BusCreator  Inputs=3
  Bus Creator1 : BusCreator  Inputs=2
  Bus Selector : BusSelector  OutputSignals=P,info.w,info.x0,info.x
  Constant1 : Constant  Value=0
  Constant2 : Constant  Value=0
  Constant3 : Constant  Value=0
  Division : Product  Inputs=*/
  Integrator : elvio/Utilities/Integrator  Ts=Ts
  Minus : Gain  Gain=-1
  Product : Product  Inputs=**
  Terminator : Terminator
  Unity : Gain
  SE : Outport
  E : Outport  Port=2
  wires:
  Minus/1 -> Unity/1  "E_store"
  Product/1 -> Integrator/1
  P/1 -> Bus Selector/1
  Bus Selector/1 -> Product/1  "<P>"
  Bus Selector/2 -> Product/2  "<w>"
  Bus Selector/4 -> Bias/1  "<x>"
  Division/1 -> SE/1
  Bus Selector/3 -> Integrator/2  "<x0>"
  Integrator/2 -> Minus/1, Division/1
  Unity/1 -> Bus Creator1/2  "energy"
  Bus Creator/1 -> Bus Creator1/1  "c"
  Bus Creator1/1 -> E/1
  Constant1/1 -> Bus Creator/1  "mass"
  Constant3/1 -> Bus Creator/3  "cost"
  Constant2/1 -> Bus Creator/2  "power"
  Bias/1 -> Division/2
  Integrator/1 -> Terminator/1

== system elvio/Basics/Split F ==
  v+ : Inport
  Freq : Inport  Port=2
  F : Inport  Port=3
  Bus Selector : BusSelector  OutputSignals=F1.Fmax,F1.Fmin,F2.Fmax,F2.Fmin
  Bus Selector1 : BusSelector  OutputSignals=Freq
  Bus v1 : BusAssignment  AssignedSignals=Freq
  Bus v2 : BusAssignment  AssignedSignals=Freq
  Range 2 : elvio/Utilities/Range
  Range 3 : elvio/Utilities/Range
  Sum1 : Sum  Inputs=+-|
  Sum2 : Sum  Inputs=|+-
  v1 : Outport
  v2 : Outport  Port=2
  wires:
  Bus v2/1 -> v2/1
  Bus v1/1 -> v1/1
  Bus Selector1/1 -> Sum2/1, Sum1/1  "<Freq>"
  v+/1 -> Bus v2/1, Bus v1/1, Bus Selector1/1
  F/1 -> Bus Selector/1
  Sum2/1 -> Bus v1/2
  Bus Selector/1 -> Range 3/1  "<Fmax>"
  Bus Selector/2 -> Range 3/3  "<Fmin>"
  Range 3/1 -> Sum1/2
  Sum1/1 -> Range 2/2
  Range 2/1 -> Sum2/2, Bus v2/2
  Bus Selector/3 -> Range 2/1  "<Fmax>"
  Bus Selector/4 -> Range 2/3  "<Fmin>"
  Freq/1 -> Range 3/2

== system elvio/Basics/Split P ==
  P1 : Inport
  E : Inport  Port=2
  Bus Assignment : BusAssignment  AssignedSignals=energy
  Bus Creator : BusCreator  Inputs=3
  Bus Creator1 : BusCreator  Inputs=2
  Bus Selector : BusSelector  OutputSignals=P,info.w,info.x0
  Bus Selector1 : BusSelector  OutputSignals=energy
  Constant1 : Constant  Value=0
  Constant2 : Constant  Value=0
  Constant3 : Constant  Value=0
  Integrator : elvio/Utilities/Integrator  Ts=Ts
  Minus : Gain  Gain=-1
  Product : Product  Inputs=**
  Sum : Sum  Inputs=-+|
  Terminator : Terminator
  Total Energy : Display
  Unity1 : Gain
  E1 : Outport
  E2 : Outport  Port=2
  wires:
  Integrator/1 -> Terminator/1
  Constant2/1 -> Bus Creator/2  "power"
  Constant3/1 -> Bus Creator/3  "cost"
  Constant1/1 -> Bus Creator/1  "mass"
  Bus Creator1/1 -> E2/1
  Bus Creator/1 -> Bus Creator1/1  "c"
  Sum/1 -> Bus Creator1/2  "energy"
  Integrator/2 -> Minus/1
  Bus Selector/3 -> Integrator/2  "<x0>"
  Bus Selector/2 -> Product/2  "<w>"
  Bus Selector/1 -> Product/1  "<P>"
  P1/1 -> Bus Selector/1
  Product/1 -> Integrator/1
  Minus/1 -> Total Energy/1, Sum/1, Unity1/1  "E_store"
  Unity1/1 -> Bus Assignment/2  "energy"
  E/1 -> Bus Selector1/1, Bus Assignment/1
  Bus Assignment/1 -> E1/1
  Bus Selector1/1 -> Sum/2  "<energy>"

== system elvio/Basics/Split v ==
  vin : Inport
  v1' : Inport  Port=2
  Bus Selector1 : BusSelector  OutputSignals=vcur,v+
  Bus v1 : BusAssignment  AssignedSignals=vcur,v+
  Bus v2 : BusAssignment  AssignedSignals=vcur,v+
  Sum1 : Sum  Inputs=-+|
  Sum5 : Sum  Inputs=-+|
  Unit Delay : UnitDelay  SampleTime=abs(Ts)
  v1 : Outport
  v2 : Outport  Port=2
  wires:
  v1'/1 -> Unit Delay/1, Sum1/1, Bus v1/3
  Sum5/1 -> Bus v2/2
  vin/1 -> Bus v2/1, Bus Selector1/1, Bus v1/1
  Bus Selector1/1 -> Sum5/2  "<vcur>"
  Bus v1/1 -> v1/1
  Bus v2/1 -> v2/1
  Sum1/1 -> Bus v2/3
  Bus Selector1/2 -> Sum1/2  "<v+>"
  Unit Delay/1 -> Bus v1/2, Sum5/1

== system elvio/Drive/Axle ==
  vreq : Inport
  Ch1 : elvio/Basics/Ch2
  Ch4 : Subsystem
  Force Loss : elvio/Basics/Force Loss  factor=factor
  Gearing : elvio/Basics/Gearing
  Radius : Constant  Value=1/radius
  Ratio1 : Constant  Value=ratio
  Wheels : elvio/Basics/Gearing
  vF : Outport
  tag scope: F=global
  wires:
  Force Loss/1 -> Ch4/1(F')
  Ch4/1(v') -> Force Loss/1
  Ch4/2(F) -> Gearing/3
  Gearing/2 -> Ch4/2(v)
  Wheels/2 -> Ch1/2
  Gearing/1 -> Ch1/1
  Force Loss/2 -> vF/1
  Wheels/1 -> [F]
  Ch1/1 -> Gearing/1
  Ratio1/1 -> Gearing/2
  [Vehicle1] -> Force Loss/2
  Ch1/2 -> Wheels/3
  Radius/1 -> Wheels/2
  vreq/1 -> Wheels/1

== system elvio/Drive/Brake ==
  vF : Inport
  Brake : elvio/Basics/Source
  Ch10 : elvio/Basics/Ch1
  Ch8 : elvio/Basics/Ch2
  Ch9 : elvio/Basics/Ch2
  Conv : elvio/Basics/Conversion
  Merge F : elvio/Basics/Merge F
  Min Torque : Constant  Value=-Tbrake
  Split F : elvio/Basics/Split F
  Terminator1 : Terminator
  Torque Limit : elvio/Basics/Set Torque Limit
  Zero : Constant  Value=0
  Zero F : Constant  Value=0
  vF' : Outport
  tag scope: F=global
  wires:
  Brake/2 -> Ch10/1
  Brake/1 -> Terminator1/1
  Zero F/1 -> Split F/2
  vF/1 -> Split F/1
  Merge F/2 -> [F]
  Conv/1 -> Ch10/2
  Ch10/1 -> Brake/1
  Ch8/1 -> Torque Limit/4
  Merge F/1 -> Split F/3
  Conv/2 -> Ch9/1
  Ch10/2 -> Conv/1
  Torque Limit/2 -> Ch8/1
  Ch9/1 -> Conv/2
  Ch9/2 -> Torque Limit/1
  Zero/1 -> Torque Limit/3
  Ch8/2 -> Merge F/1
  Min Torque/1 -> Torque Limit/2
  Split F/1 -> Ch8/2
  Torque Limit/1 -> Ch9/2
  Split F/2 -> vF'/1
  [Vehicle1] -> Merge F/2

== system elvio/Drive/Bus ==
  P1 : Inport
  P2 : Inport  Port=2
  Merge P : elvio/Basics/Merge P
  Split P : elvio/Basics/Split P
  P : Outport
  tag scope: E2=global, F=global
  wires:
  [E] -> Split P/2
  Merge P/1 -> P/1
  P1/1 -> Merge P/1
  Split P/1 -> [F]
  P2/1 -> Merge P/2
  Merge P/2 -> Split P/1
  Split P/2 -> [E2]

== system elvio/Drive/Clutch ==
  vF : Inport
  Brake : elvio/Basics/Source
  Bus Selector : BusSelector  OutputSignals=v+
  Ch10 : elvio/Basics/Ch1
  Ch9 : elvio/Basics/Ch2
  Conv : elvio/Basics/Conversion
  Merge v : elvio/Basics/Merge v
  MinMax : MinMax  Function=max  Inputs=2
  Speed : Constant  Value=speed
  Split v : elvio/Basics/Split v
  Terminator1 : Terminator
  vF' : Outport
  tag scope: F=global
  wires:
  [Vehicle1] -> Merge v/1
  Split v/1 -> vF'/1
  Ch9/1 -> Conv/2
  Ch10/2 -> Conv/1
  Conv/2 -> Ch9/1
  Ch10/1 -> Brake/1
  Conv/1 -> Ch10/2
  Merge v/1 -> [F]
  vF/1 -> Bus Selector/1, Split v/1
  Brake/1 -> Terminator1/1
  Brake/2 -> Ch10/1
  Split v/2 -> Ch9/2
  Ch9/2 -> Merge v/2
  MinMax/1 -> Split v/2
  Speed/1 -> MinMax/2
  Bus Selector/1 -> MinMax/1  "<v+>"

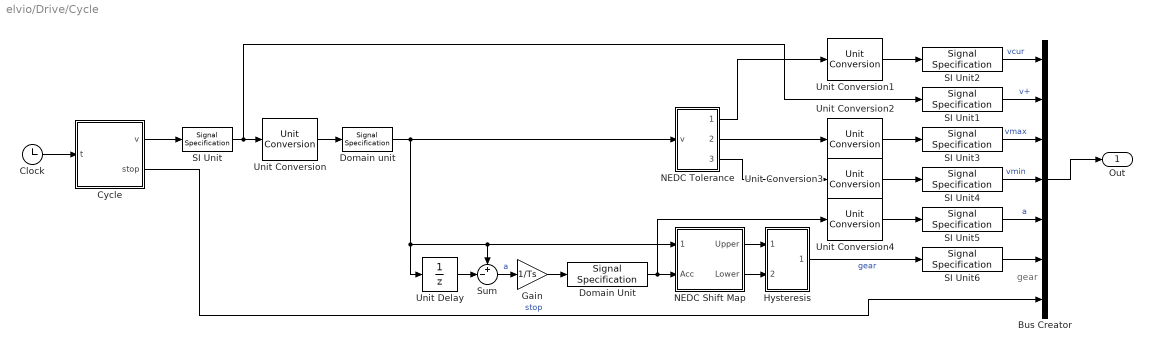
== system elvio/Drive/Cycle ==
  note: gear
  Bus Creator : BusCreator  Inputs=7
  Clock : Clock
  Cycle : Subsystem  mask{data=eval(data)}
      mask prompts: data "Cycle data:"
  Domain Unit : SignalSpecification  Unit=km/(h*s)
  Domain unit : SignalSpecification  Unit=km/h
  Gain : Gain  Gain=1/Ts
  Hysteresis : Subsystem
  NEDC Shift Map : Subsystem
  NEDC Tolerance : Subsystem
  SI Unit{,1..4} (5 alike) : SignalSpecification  Unit=m/s
  SI Unit5 : SignalSpecification  Unit=m/s^2
  SI Unit6 : SignalSpecification  Unit=1
  Sum : Sum  Inputs=+-|
  Unit Conversion{,1..4} (5 alike) : UnitConversion
  Unit Delay : UnitDelay  SampleTime=-1
  Out : Outport
  wires:
  NEDC Shift Map/1(Upper) -> Hysteresis/1(Max)
  NEDC Shift Map/2(Lower) -> Hysteresis/2(Min)
  Unit Conversion/1 -> Domain unit/1
  Domain unit/1 -> NEDC Tolerance/1(v), Sum/1, NEDC Shift Map/1(Speed), Unit Delay/1
  Unit Delay/1 -> Sum/2
  SI Unit4/1 -> Bus Creator/4  "vmin"
  Sum/1 -> Gain/1  "a"
  SI Unit1/1 -> Bus Creator/2  "v+"
  SI Unit3/1 -> Bus Creator/3  "vmax"
  Hysteresis/1(gear) -> SI Unit6/1  "gear"
  Bus Creator/1 -> Out/1
  SI Unit2/1 -> Bus Creator/1  "vcur"
  NEDC Tolerance/1(Delay) -> Unit Conversion1/1
  NEDC Tolerance/2(Upper) -> Unit Conversion2/1
  NEDC Tolerance/3(Lower) -> Unit Conversion3/1
  SI Unit5/1 -> Bus Creator/5  "a"
  Unit Conversion1/1 -> SI Unit2/1
  SI Unit/1 -> SI Unit1/1, Unit Conversion/1
  Unit Conversion2/1 -> SI Unit3/1
  Unit Conversion3/1 -> SI Unit4/1
  Unit Conversion4/1 -> SI Unit5/1
  Gain/1 -> Domain Unit/1
  Domain Unit/1 -> NEDC Shift Map/2(Acc), Unit Conversion4/1
  SI Unit6/1 -> Bus Creator/6
  Cycle/2(stop) -> Bus Creator/7  "stop"
  Clock/1 -> Cycle/1(t)
  Cycle/1(v) -> SI Unit/1

== system elvio/Drive/Dyno ==
  Bus Creator1 : BusCreator  Inputs=4
  Bus Creator2 : BusCreator  Inputs=4
  Bus Selector : BusSelector  OutputSignals=Fmax,Fmin
  Constant1 : Constant  Value=speed
  Constant2 : Constant  Value=request
  Divide : Product  Inputs=/*
  Manual Switch : ManualSwitch  CurrentSetting=0
  Range : elvio/Utilities/Range
  To Workspace1 : ToWorkspace  VariableName=torque  SampleTime=-1
      settings: MaxDataPoints=1
  Ts : Constant  Value=Ts
  Unity1 : Gain
  Unity2 : Gain
  Weight : Constant
  Zero1 : Gain  Gain=0
  Zero4 : Gain
  vF : Outport
  wires:
  Divide/1 -> Manual Switch/1
  Bus Selector/1 -> Range/1  "<Fmax>"
  Zero1/1 -> Bus Creator2/4  "x0"
  Weight/1 -> Bus Creator2/1  "w"
  Bus Selector/2 -> Range/3  "<Fmin>"
  Ts/1 -> Bus Creator2/2  "Ts"
  Zero4/1 -> Bus Creator2/3  "x"
  Constant2/1 -> Divide/2, Manual Switch/2
  [Dyno1] -> Bus Selector/1
  Unity2/1 -> Bus Creator1/3  "v+"
  Manual Switch/1 -> Range/2
  Bus Creator2/1 -> Bus Creator1/1  "info"
  Range/1 -> Bus Creator1/4, To Workspace1/1  "Freq"
  Bus Creator1/1 -> vF/1
  Unity1/1 -> Bus Creator1/2  "vcur"
  Constant1/1 -> Divide/1, Unity1/1, Unity2/1, Zero1/1, Zero4/1

== system elvio/Drive/EUCycle ==
  Bias : Bias  Bias=+2
  Bias1 : Bias  Bias=-2
  Bus Creator : BusCreator  Inputs=7
  Clock : Clock
  NEDC : Subsystem  mask{data=eval(data)}
      mask prompts: data "Cycle Data:"
  Signal Specification1 : SignalSpecification  Unit=m/s
  Signal Specification2 : SignalSpecification  Unit=m/s
  Signal Specification3 : SignalSpecification  Unit=m/s
  Signal Specification4 : SignalSpecification  Unit=km/hr
  Signal Specification5 : SignalSpecification  Unit=km/hr
  Todo : Constant  Value=0
  Unit Conversion : UnitConversion
  Unit Conversion1 : UnitConversion
  Unit Conversion2 : UnitConversion
  Unit Delay : UnitDelay  SampleTime=-1
  Out : Outport
  wires:
  Bus Creator/1 -> Out/1
  Clock/1 -> NEDC/1(t)
  NEDC/1(v) -> Unit Conversion/1, Bias/1, Bias1/1  "v"
  Bias/1 -> Signal Specification4/1  "vmax"
  Bias1/1 -> Signal Specification5/1  "vmin"
  Signal Specification1/1 -> Bus Creator/3  "vmax"
  Signal Specification2/1 -> Bus Creator/4  "vmin"
  Signal Specification3/1 -> Bus Creator/2, Unit Delay/1  "v+"
  Unit Conversion/1 -> Signal Specification3/1
  Unit Conversion1/1 -> Signal Specification1/1
  Unit Conversion2/1 -> Signal Specification2/1
  NEDC/2(g) -> Bus Creator/6  "gear"
  Todo/1 -> Bus Creator/5  "a"
  Unit Delay/1 -> Bus Creator/1  "vcur"
  Signal Specification4/1 -> Unit Conversion1/1
  Signal Specification5/1 -> Unit Conversion2/1
  NEDC/3(stop) -> Bus Creator/7  "stop"

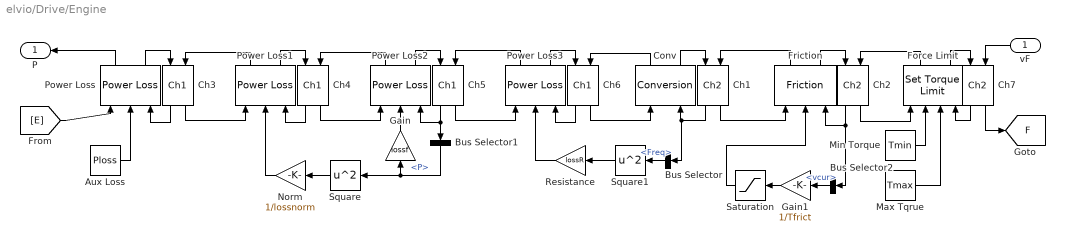
== system elvio/Drive/Engine ==
  vF : Inport
  Aux Loss : Constant  Value=Ploss
  Bus Selector : BusSelector  OutputSignals=Freq
  Bus Selector1 : BusSelector  OutputSignals=P
  Bus Selector2 : BusSelector  OutputSignals=vcur
  Ch1 : elvio/Basics/Ch2
  Ch2 : elvio/Basics/Ch2
  Ch{3..6} (4 alike) : elvio/Basics/Ch1
  Ch7 : elvio/Basics/Ch2
  Conv : elvio/Basics/Conversion
  Force Limit : elvio/Basics/Set Torque Limit
  Friction : elvio/Basics/Friction
  Gain : Gain  Gain=lossf
  Gain1 : Gain  Gain=1/Tfrict
  Max Tqrue : Constant  Value=Tmax
  Min Torque : Constant  Value=Tmin
  Norm : Gain  Gain=1/lossnorm
  Power Loss{,1..3} (4 alike) : elvio/Basics/Power Loss
  Resistance : Gain  Gain=lossR
  Saturation : Saturate  UpperLimit=Tfrict  LowerLimit=-Tfrict  ZeroCross=off
  Square : Math  Operator=square  SaturateOnIntegerOverflow=on
  Square1 : Math  Operator=square  SaturateOnIntegerOverflow=on
  P : Outport
  tag scope: F=global
  wires:
  Saturation/1 -> Friction/2
  Ch7/1 -> Force Limit/4
  Friction/2 -> Ch2/1
  Aux Loss/1 -> Power Loss/2
  Max Tqrue/1 -> Force Limit/3
  Force Limit/1 -> Ch2/2
  Ch2/1 -> Bus Selector2/1, Friction/3
  Ch2/2 -> Force Limit/1
  Power Loss/1 -> P/1
  Power Loss/2 -> Ch3/1
  Ch3/1 -> Power Loss/3
  Conv/2 -> Ch1/1
  Friction/1 -> Ch1/2
  Ch1/2 -> Friction/1
  Ch1/1 -> Bus Selector/1, Conv/2
  [E] -> Power Loss/1
  Ch3/2 -> Power Loss1/1
  Ch4/1 -> Power Loss1/3
  Power Loss1/2 -> Ch4/1
  Power Loss1/1 -> Ch3/2
  Power Loss2/1 -> Ch4/2
  Power Loss2/2 -> Ch5/1
  Ch5/1 -> Bus Selector1/1, Power Loss2/3
  Ch4/2 -> Power Loss2/1
  Bus Selector1/1 -> Square/1, Gain/1  "<P>"
  Gain/1 -> Power Loss2/2
  Norm/1 -> Power Loss1/2
  Square/1 -> Norm/1
  Square1/1 -> Resistance/1
  Ch5/2 -> Power Loss3/1
  Ch6/1 -> Power Loss3/3
  Power Loss3/2 -> Ch6/1
  Power Loss3/1 -> Ch5/2
  Conv/1 -> Ch6/2
  Ch6/2 -> Conv/1
  Bus Selector/1 -> Square1/1  "<Freq>"
  Resistance/1 -> Power Loss3/2
  Ch7/2 -> [F]
  vF/1 -> Ch7/2
  Force Limit/2 -> Ch7/1
  Min Torque/1 -> Force Limit/2
  Gain1/1 -> Saturation/1
  Bus Selector2/1 -> Gain1/1  "<vcur>"
